simulink model "sample_simulink"  (R2020b)
settings: Solver=FixedStepDiscrete  StartTime=0.0  StopTime=inf  FixedStep=0.02  RelTol=1e-3
undefined symbols (not defined in the file): Serial_Port, Standard_Devices
libraries: sldrtlib x1
settings Model: Creator=Admin  LastModifiedBy=Duncan

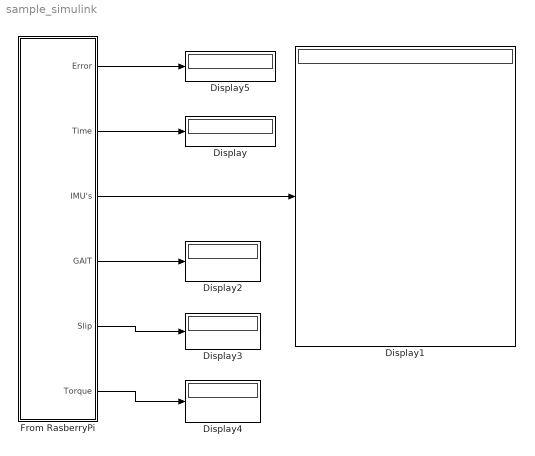
== system sample_simulink ==
  Display{,1..5} (6 alike) : Display
  From RasberryPi : Subsystem
  wires:
  From RasberryPi/2(Time) -> Display/1
  From RasberryPi/3(IMU's) -> Display1/1
  From RasberryPi/4(GAIT) -> Display2/1
  From RasberryPi/5(Slip) -> Display3/1
  From RasberryPi/6(Torque) -> Display4/1
  From RasberryPi/1(Error) -> Display5/1

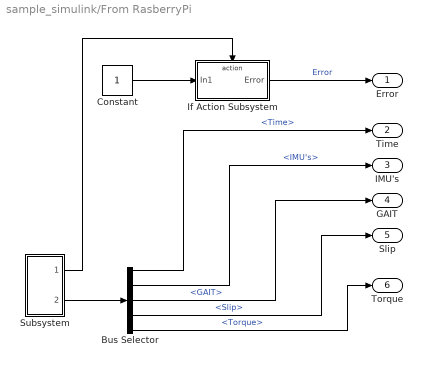
== system sample_simulink/From RasberryPi ==
  Bus Selector : BusSelector  OutputSignals=Time,IMU's,GAIT,Slip,Torque
  Constant : Constant
  If Action Subsystem : Subsystem  TreatAsAtomicUnit=on
  Subsystem : Subsystem
  Error : Outport
  Time : Outport  Port=2
  IMU's : Outport  Port=3
  GAIT : Outport  Port=4
  Slip : Outport  Port=5
  Torque : Outport  Port=6
  wires:
  Constant/1 -> If Action Subsystem/1(In1)
  Subsystem/1(Error) -> If Action Subsystem/Action
  If Action Subsystem/1(Error) -> Error/1  "Error"
  Subsystem/2(Data) -> Bus Selector/1
  Bus Selector/1 -> Time/1  "<Time>"
  Bus Selector/2 -> IMU's/1  "<IMU's>"
  Bus Selector/3 -> GAIT/1  "<GAIT>"
  Bus Selector/4 -> Slip/1  "<Slip>"
  Bus Selector/5 -> Torque/1  "<Torque>"

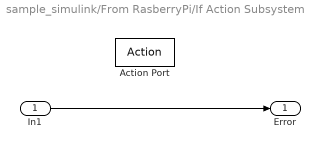
== system sample_simulink/From RasberryPi/If Action Subsystem ==
  In1 : Inport
  Action Port : ActionPort  ActionPortLabel=else
  Error : Outport
  wires:
  In1/1 -> Error/1

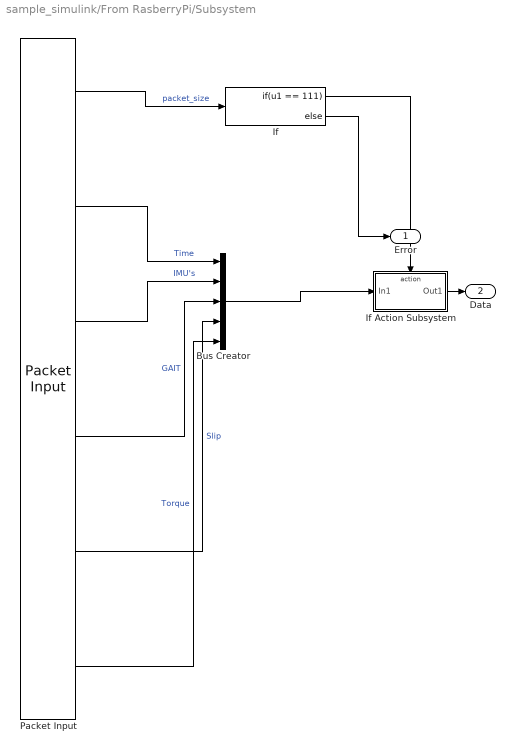
== system sample_simulink/From RasberryPi/Subsystem ==
  Bus Creator : BusCreator  Inputs=5
  If : If  IfExpression=u1 == 111
  If Action Subsystem : Subsystem  TreatAsAtomicUnit=on
  Packet Input : sldrtlib/Packet Input  SampleTime=-1  MaxMissedTicks=inf  ShowMissedTicks=off  YieldWhenWaiting=on  DrvName=Standard_Devices/Serial_Port  DrvAddress=6  DrvOptions=[115200 8 0 0 0 0 0 0]  PacketSize=111  DataTypes={'uint8' , 'single' , '49*int16', '2*int8', '2*int16','int16'}  ShowReady=off  ShowError=off  PacketID=1  ByteOrder=1  ShowTimestamp=off
      settings: AttributesFormatString=Serial Port [6]
  Error : Outport
  Data : Outport  Port=2
  wires:
  If/1 -> If Action Subsystem/Action
  If Action Subsystem/1(Out1) -> Data/1
  If/2 -> Error/1
  Packet Input/1 -> If/1  "packet_size"
  Packet Input/2 -> Bus Creator/1  "Time"
  Packet Input/3 -> Bus Creator/2  "IMU's"
  Packet Input/4 -> Bus Creator/3  "GAIT"
  Packet Input/5 -> Bus Creator/4  "Slip"
  Bus Creator/1 -> If Action Subsystem/1(In1)
  Packet Input/6 -> Bus Creator/5  "Torque"

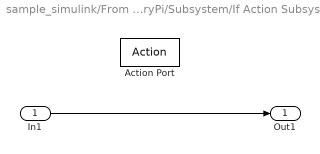
== system sample_simulink/From RasberryPi/Subsystem/If Action Subsystem ==
  In1 : Inport
  Action Port : ActionPort  ActionPortLabel=if(u1 == 111)
  Out1 : Outport
  wires:
  In1/1 -> Out1/1
